simulink model "mrac_model3"  (R2022a)
settings: Solver=VariableStepAuto  StartTime=0.0  StopTime=100  RelTol=1e-3
values from neighbouring files (symbols this model uses):
  params = getParamsMRAC(0.25, 1, 10e-3, 10e-5, 100)    [mrac.m]
libraries: slctrlblks x1
settings Model: Creator=mateusz  LastModifiedBy=mateusz

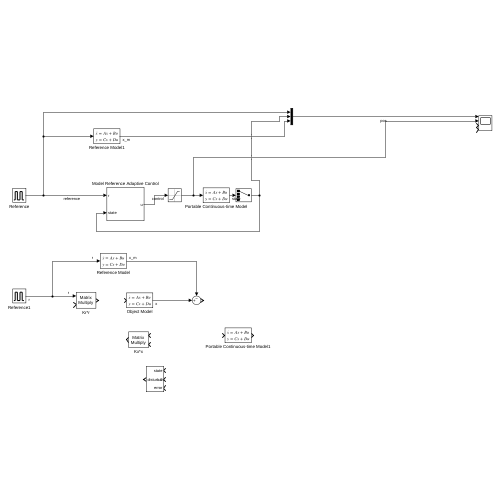
[thumbnail: Simulink's stored preview of the top-level diagram]
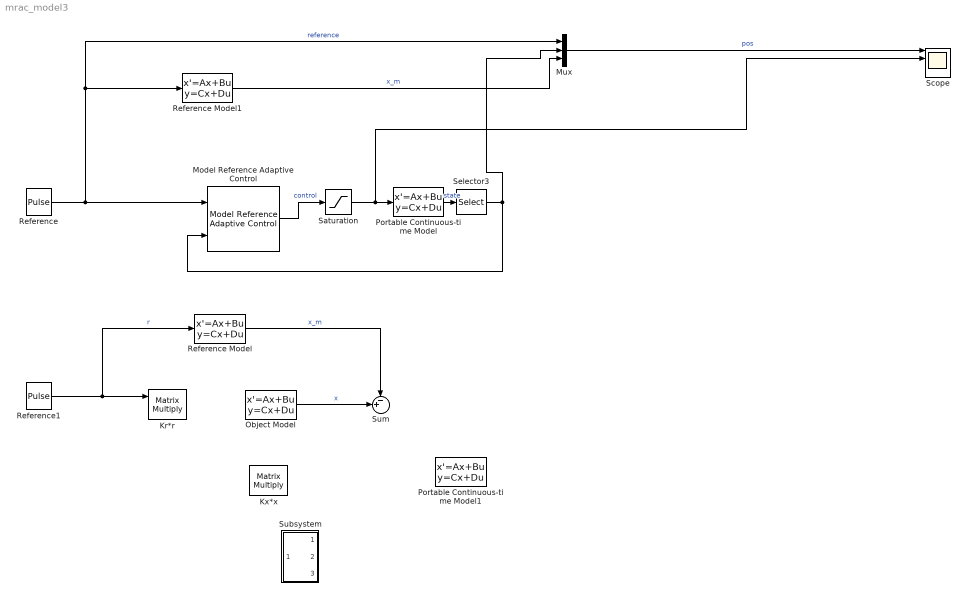
== system mrac_model3 ==
  Kr*r : Product  Multiplication=Matrix(*)
  Kx*x : Product  Multiplication=Matrix(*)
  Model Reference Adaptive Control : slctrlblks/Model Reference Adaptive Control  selectType=Direct  A=params.Am  B=params.Bm  Ahat=0  ALrEnable=on  gamma_a=1  ALrEnableMod=on  Bhat=1  BLrEnable=on  gamma_b=1  BLrEnableMod=on  externalKtauEnable=off  k_tau=-1  estParamOutput=off  Am=params.Am  Bm=params.Bm  kx=params.Kx  FBLrEnable=on  gamma_kx=params.gamma_x  FBLrEnableMod=on  kr=params.Kr  FFLrEnable=off  gamma_kr=1  FFLrEnableMod=off  AdaptEnable=off  gamma=params.gamma_w  WLrEnableMod=off  Q=max(max(params.Q))  FeatureTypeOptions=State  nCen=20  cSpanMin=-1  cSpanMax=1  cSig=5  adaptiveCntrlOutport=off  modChoice=None  sigma_val=0.1
      settings: SourceProductBaseCode=SD
  Mux : Mux  Inputs=3
  Object Model : StateSpace  A=|  B=[0;0;0;2.59e4];  C=eye(4,4)  D=zeros(4,1)  InitialCondition=0
      | [0  1  0    0;
      |      0 -5  4.5  0;
      |      0  0 -0.7108*2  2*23.6012;
      |      0  0 -5.3898 -4040];
  Portable Continuous-time Model : StateSpace  A=|  B=[0;0;0;2.59e4];  C=eye(4,4)  D=zeros(4,1)  InitialCondition=0
      | [0  1  0    0;
      |      0 -5  4.5  0;
      |      0  0 -0.7108*2  2*23.6012;
      |      0  0 -5.3898 -4040];
  Portable Continuous-time Model1 : StateSpace  A=|  B=[0;0;0;2.59e4];  C=eye(4,4)  D=zeros(4,1)  InitialCondition=0
      | [0  1  0    0;
      |      0 -5  4.5  0;
      |      0  0 -0.7108*2  2*23.6012;
      |      0  0 -5.3898 -4040];
  Reference : DiscretePulseGenerator  PulseType=Time based  Amplitude=6.28*25  Period=20  PulseWidth=50
  Reference Model : StateSpace  InitialCondition=0
  Reference Model1 : StateSpace  A=params.Am  B=params.Bm  D=0  InitialCondition=0
  Reference1 : DiscretePulseGenerator  PulseType=Time based  Period=10  PulseWidth=50
  Saturation : Saturate  UpperLimit=1  LowerLimit=-1
  Scope : Scope  NumInputPorts=4
  Selector3 : Selector  InputPortWidth=4  IndexOptions=Index vector (dialog)  Indices=[1]  OutputSizes=1
  Subsystem : Subsystem
  Sum : Sum  Inputs=-+|
  wires:
  Model Reference Adaptive Control/1 -> Saturation/1  "control"
  Reference/1 -> Reference Model1/1, Mux/1, Model Reference Adaptive Control/1  "reference"
  Selector3/1 -> Mux/2, Model Reference Adaptive Control/2
  Mux/1 -> Scope/1  "pos"
  Reference1/1 -> Reference Model/1, Kr*r/1  "r"
  Reference Model/1 -> Sum/1  "x_m"
  Object Model/1 -> Sum/2  "x"
  Reference Model1/1 -> Mux/3  "x_m"
  Saturation/1 -> Scope/2, Portable Continuous-time Model/1
  Portable Continuous-time Model/1 -> Selector3/1  "state"

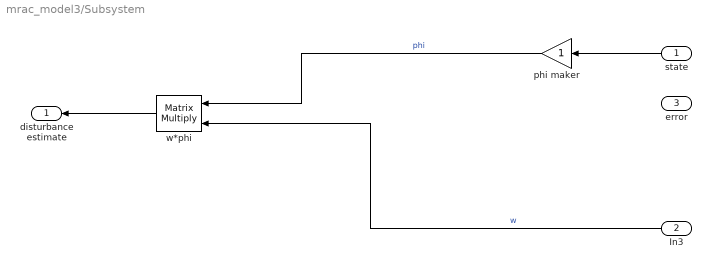
== system mrac_model3/Subsystem ==
  state : Inport
  In3 : Inport  Port=2
  error : Inport  Port=3
  phi maker : Gain
  w*phi : Product  Multiplication=Matrix(*)
  disturbance estimate : Outport
  wires:
  w*phi/1 -> disturbance estimate/1
  In3/1 -> w*phi/2  "w"
  state/1 -> phi maker/1
  phi maker/1 -> w*phi/1  "phi"
